simulink model "nonlinear"  (Simulink 7.7)
settings: Solver=ode45  StartTime=0.0  StopTime=10  RelTol=1e-3
values from neighbouring files (symbols this model uses):
  b1 = Vin/L    (= 800000)    [nonlinearcommande.m]
  f11 = (-1/L)*(RL+RS/4)    (= -5653.33333333)    [nonlinearcommande.m]
  f22 = -1/(R*C)    (= -1063.82978723)    [nonlinearcommande.m]
  g12 = -1/L    (= -66666.6666667)    [nonlinearcommande.m]
  g21 = 1/C    (= 106382.978723)    [nonlinearcommande.m]
undefined symbols (not defined in the file or in its folder): sgn
libraries: simulink x1
settings Model: Creator=etudiants  LastModifiedBy=Nicolas
settings OptimizationCC: InitFltsAndDblsToZero=on
settings DebuggingCC: StrictBusMsg=Warning

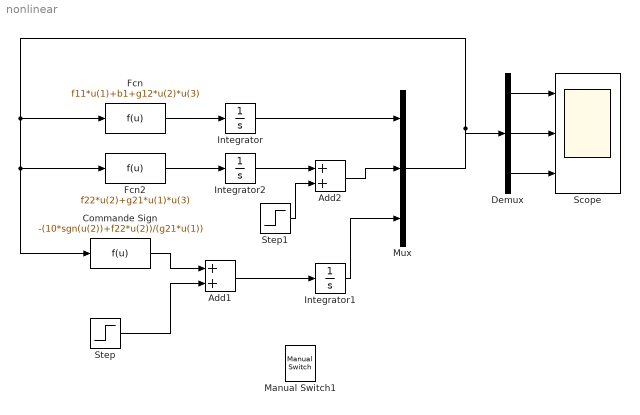
== system nonlinear ==
  Add1 : Sum
  Add2 : Sum
  Commande Sign : Fcn  Expr=-(10*sgn(u(2))+f22*u(2))/(g21*u(1))
  Demux : Demux  Outputs=3
  Fcn : Fcn  Expr=f11*u(1)+b1+g12*u(2)*u(3)
  Fcn2 : Fcn  Expr=f22*u(2)+g21*u(1)*u(3)
  Integrator : Integrator  InitialCondition=0.5
  Integrator1 : Integrator  InitialCondition=0.5
  Integrator2 : Integrator  InitialCondition=0.5
  Manual Switch1 : simulink/Signal Routing/Manual Switch  SystemSampleTime=-1  sw=0  action=0  varsize=off
  Mux : Mux  Inputs=3
  Scope : Scope  NumInputPorts=3
      settings: YMin=141.36~-1~-1  YMax=141.5~1~1
  Step : Step  After=0.5  SampleTime=0
  Step1 : Step  After=0.5  SampleTime=0
  wires:
  Fcn/1 -> Integrator/1
  Demux/1 -> Scope/1
  Demux/2 -> Scope/2
  Fcn2/1 -> Integrator2/1
  Mux/1 -> Fcn/1, Fcn2/1, Commande Sign/1, Demux/1
  Demux/3 -> Scope/3
  Integrator/1 -> Mux/1
  Step/1 -> Add1/2
  Commande Sign/1 -> Add1/1
  Integrator1/1 -> Mux/3
  Add1/1 -> Integrator1/1
  Integrator2/1 -> Add2/1
  Add2/1 -> Mux/2
  Step1/1 -> Add2/2
